simulink model "pidinfuzzylookup"  (Simulink 7.6)
settings: Solver=ode45  StartTime=0.0  StopTime=20  RelTol=1e-3
settings Model: Creator=kif  LastModifiedBy=kif

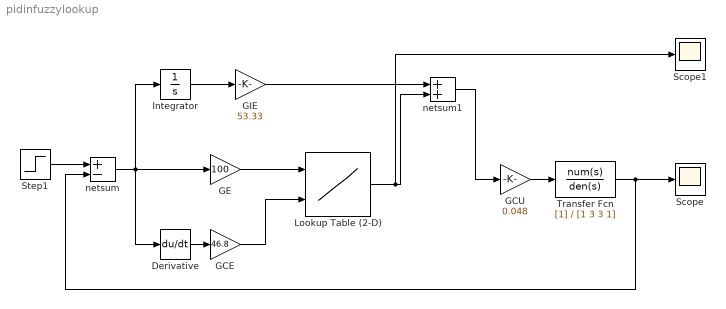
== system pidinfuzzylookup ==
  Derivative : Derivative
  GCE : Gain  Gain=46.8
  GCU : Gain  Gain=0.048
  GE : Gain  Gain=100
  GIE : Gain  Gain=53.33
  Integrator : Integrator
  Lookup Table (2-D) : Lookup2D  RowIndex=[1:5]  ColumnIndex=[1:5]  Table="[-187.8 -143.6 -93.9 -44.2 0.0;-143.6 -99.3 -49.6  0.0  44.2;-93.9  -49.6  0.0 49.6 93.9;-44.2 0.0 49.6 99.3 143.6;0.0 44.2 93.9 143.6 187.8]"
  Scope : Scope
  Scope1 : Scope
      settings: TimeRange=20  YMin=-70  YMax=100
  Step1 : Step  SampleTime=0
  Transfer Fcn : TransferFcn  Denominator=[1 3 3 1]
  netsum : Sum  Inputs=+-  SaturateOnIntegerOverflow=on  InputSameDT=on  OutDataTypeStr=Inherit: Same as first input
  netsum1 : Sum  Inputs=2  SaturateOnIntegerOverflow=on  InputSameDT=on  OutDataTypeStr=Inherit: Same as first input
  wires:
  netsum/1 -> Integrator/1, Derivative/1, GE/1
  Derivative/1 -> GCE/1
  Integrator/1 -> GIE/1
  Lookup Table (2-D)/1 -> netsum1/2, Scope1/1
  netsum1/1 -> GCU/1
  Transfer Fcn/1 -> Scope/1, netsum/2
  GIE/1 -> netsum1/1
  GE/1 -> Lookup Table (2-D)/1
  GCE/1 -> Lookup Table (2-D)/2
  GCU/1 -> Transfer Fcn/1
  Step1/1 -> netsum/1
